simulink model "ad9361_rx_rates"  (R2017b)
settings: Solver=ode23  StartTime=0.0  StopTime=inf  RelTol=1e-3  EnableMultiTasking=on
PreLoadFcn:
  | SampleTime_rx = 1.302083333333333334e-7;
  | 
  | ad9361_preload(bdroot,'rx')
undefined symbols (not defined in the file or in its folder): magnitude, var
libraries: dspsrcs4 x8, dspmathops x6, dsparch4 x4, ad9361_models x1
CloseFcn:
  | clear ad9361_rx_hm1Filt ad9361_rx_hm2Filt;
  | clear ad9361_rx_hm3Filt ad9361_rx_hm4Filt;
  | clear SampleTime_rx;
settings Model: Creator=The MathWorks Inc.  LastModifiedBy=ppradhan
settings DataIOCC: ExternalInput=txWaveform  SaveFormat=StructureWithTime  SaveOutput=off  SignalLogging=off  DSMLogging=off  SaveTime=off  OutputSaveName=rx
settings OptimizationCC: DefaultParameterBehavior=Inlined  InlineInvariantSignals=on  EfficientMapNaN2IntZero=off  LifeSpan=inf  SimCompilerOptimization=on
settings DebuggingCC: ReadBeforeWriteMsg=DisableAll  WriteAfterWriteMsg=DisableAll  WriteAfterReadMsg=DisableAll  UnderspecifiedInitializationDetection=Classic  MergeDetectMultiDrivingBlocksExec=none  SolverPrmCheckMsg=warning  InheritedTsInSrcMsg=none  MultiTaskDSMMsg=none  IntegerOverflowMsg=none  AllowSymbolicDim=off  SFUnexpectedBacktrackingDiag=warning  SFNoUnconditionalDefaultTransitionDiag=none  SFUndirectedBroadcastEventsDiag=none  SFExecutionAtInitializationDiag=none  IntegerSaturationMsg=none
settings HardwareCC: ProdBitPerPointer=32  ProdBitPerSizeT=32  ProdBitPerPtrDiffT=32  ProdLargestAtomicFloat=None  ProdIntDivRoundTo=Undefined  ProdEndianess=Unspecified  ProdWordSize=32  ProdHWDeviceType=32-bit Generic  TargetBitPerPointer=64  TargetBitPerSizeT=64  TargetBitPerPtrDiffT=64  TargetLongLongMode=on  TargetIntDivRoundTo=Zero  TargetEndianess=LittleEndian  TargetWordSize=64  TargetHWDeviceType=MATLAB Host  ProdEqTarget=off
settings ModelReferenceCC: UpdateModelReferenceTargets=IfOutOfDate  PropagateSignalLabelsOutOfModel=off
settings SFSimCC: SFSimEcho=off
settings CodeAppCC: MaxIdLength=128  StateflowObjectComments=on
settings GRTTargetCC: TargetLangStandard=C89/C90 (ANSI)  GeneratePreprocessorConditionals=Disable all  CombineOutputUpdateFcns=off  GRTInterface=on
settings ConfigComp: CovMetricSettings=dw  CovHtmlReporting=on  CovSaveCumulativeToWorkspaceVar=on  CovSaveSingleToWorkspaceVar=on  CovExternalEMLEnable=off  CovSFcnEnable=off
settings SimscapeCC: ExplicitSolverDiagnosticOptions=none

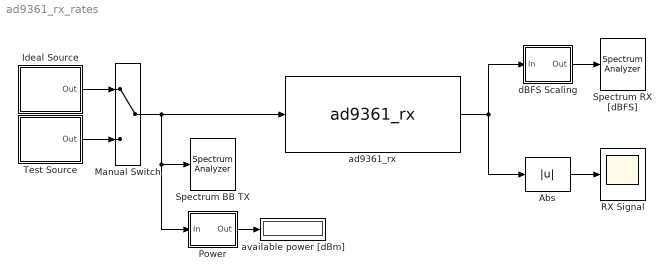
== system ad9361_rx_rates ==
  Abs : Abs
  Ideal Source : Subsystem  mask{Sel=Single CW tone, CW=1e6, Pow=-70, Tstep=1.302083333333333e-07, Ovs=4}
      mask prompts: Sel "Select source"; CW "Frequency (Hz)"; Pow "Power (dBm)"; Tstep "Sample time (s)"; Ovs "Oversampling"
      mask TypeOptions Sel: CW + 1MHz tone | Single CW tone | Dual CW tone
      mask DialogControl DescGroupVar Prompt: Ideal Test Source
  Manual Switch : ManualSwitch
  "Power  " : Subsystem  mask{R=50}
      mask prompts: R "Reference Impedance [Ohm]"
      mask DialogControl DescGroupVar Prompt: Power Meter
  RX Signal : Scope
  Spectrum BB TX : SpectrumAnalyzer
  Spectrum RX [dBFS] : SpectrumAnalyzer
  Test Source : Subsystem  mask{TestSigType=5MHz LTE-like test signal, RxCustVector=complex(rand(1000,1), rand(1000,1)), Tstep=1.302083333333333e-07, OverSample=4, LTE_Pow=-50, hasBlockerCW=off, CW_Blocker_Freq=3e6, CW_Blocker_Pow=-20, hasBlockerLTE=off, LTE_Blocker_OffsetFreq=3e6, LTE_Blocker_Pow=-30}
      mask prompts: TestSigType "Test signal"; RxCustVector "Custom test vector complex data (I, Q)"; Tstep "Sample time (s)"; OverSample "Oversampling"; LTE_Pow "Power (dBm)"; hasBlockerCW "CW blocker"; CW_Blocker_Freq "Frequency CW blocker (Hz)"; CW_Blocker_Pow "Power CW blocker (dBm)"; hasBlockerLTE "LTE-like blocker"; LTE_Blocker_OffsetFreq "Frequency offset LTE-like blocker (Hz)"; LTE_Blocker_Pow "Power LTE-like blocker (dBm)"
      mask init:
      | load ad9361_LTE_data;
      | load ad9361_LTE_blocker;
      | 
      | if strcmpi(TestSigType,'5MHz LTE-like test signal')
      |     tx = tx5;
      |     tx_bl = tx5_bl;
      |     SampleTime_rx = 1/info5.SamplingRate;
      |     LTE = 5;
      | elseif strcmpi(TestSigType,'10MHz LTE-like test signal')
      |     tx = tx10;
      |     tx_bl = tx10_bl;
      |     LTE = 10;
      |     SampleTime_rx = 1/info10.SamplingRate;
      | elseif strcmpi(TestSigType,'20MHz LTE-like test signal')
      |     tx = tx20;
      |     tx_bl = tx20_bl;
      |     LTE = 20;
      |     SampleTime_rx = 1/info20.SamplingRate;
      | elseif strcmpi(TestSigType,'Custom Signal (LTE blocker NOT allowed)')
      |     LTE = 0;
      |     tx = RxCustVector;
      |     tx_bl = RxCustVector;
      |     SampleTime_rx = str2num(get_param(gcb,'Tstep'));
      | else
      |     error(message('simrf:simrfad9361:UnknownTestSig',gcb,TestSigType));
      | end
      | 
      | if ~any(strcmpi(get_param(bdroot(gcb), 'SimulationStatus'),             ...
      |             {'running' 'paused'}))
      |   set_param(gcb,'Tstep',num2str(SampleTime_rx,16));
      |   idlSrc = [bdroot '/Ideal Source'];
      |   set_param(idlSrc,'Tstep',num2str(SampleTime_rx,16));
      |   if ~strcmp(TestSigType,'Custom signal (LTE blocker NOT allowed)')
      |     assignin('base', 'SampleTime_rx', SampleTime_rx);
      |   end
      |   p = Simulink.Mask.get(gcb);
      |   p.Parameters(3).Value = num2str(SampleTime_rx,16);
      | end
      mask TypeOptions TestSigType: 5MHz LTE-like test signal | 10MHz LTE-like test signal | 20MHz LTE-like test signal | Custom Signal (LTE blocker NOT allowed)
      mask Callback TestSigType:
      | % Set Mask visibilites and enables
      | ad9361_rx_mask_callbacks(gcb,'TestSigType')
      mask Callback hasBlockerCW:
      | % Set Mask visibilites and enables
      | ad9361_rx_mask_callbacks(gcb,'hasBlockerCW')
      mask Callback hasBlockerLTE:
      | % Set Mask visibilites and enables
      | ad9361_rx_mask_callbacks(gcb,'hasBlockerLTE')
      mask DialogControl DescGroupVar Prompt: Test Source RX
  ad9361_rx : ad9361_models/ad9361_rx  TestSignal=5MHz LTE  LO=2e9  RF=2e9  Trf=1/(4*7.68e6)
      settings: SourceProductName=RF Blockset Models for Analog Devices RF Transceivers
  available power [dBm] : Display
  dBFS Scaling : Subsystem
  wires:
  Test Source/1(Out) -> Manual Switch/2
  Ideal Source/1(Out) -> Manual Switch/1
  Manual Switch/1 -> ad9361_rx/1, Spectrum BB TX/1, "Power  "/1(In)
  "Power  "/1(Out) -> available power [dBm]/1
  dBFS Scaling/1(Out) -> Spectrum RX [dBFS]/1
  ad9361_rx/1 -> Abs/1, dBFS Scaling/1(In)
  Abs/1 -> RX Signal/1

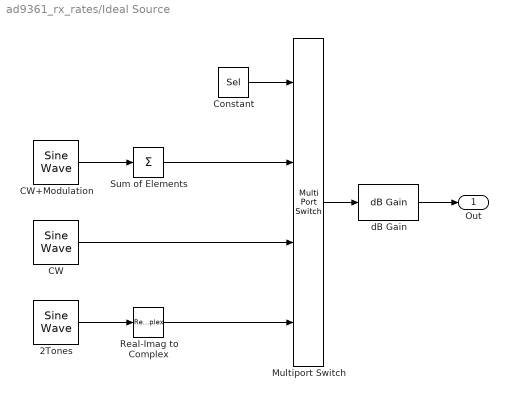
== system ad9361_rx_rates/Ideal Source ==
  2Tones : dspsrcs4/Sine Wave  Amplitude=sqrt(2)  Frequency=CW/2  Phase=0  SampleMode=Discrete  OutComplex=Real  CompMethod=Trigonometric fcn  TableSize=Speed  SampleTime=Tstep/Ovs  SamplesPerFrame=1  ResetState=Restart at time zero  OutputFrames=on  dataType=double  wordLen=16  udDataType=sfix(16)  fracBitsMode=Best precision  numFracBits=15  OutDataTypeStr=double  LastOutDataTypeStr=double
  CW : dspsrcs4/Sine Wave  Amplitude=1  Frequency=CW  Phase=0  SampleMode=Discrete  OutComplex=Complex  CompMethod=Trigonometric fcn  TableSize=Speed  SampleTime=Tstep/Ovs  SamplesPerFrame=1  ResetState=Restart at time zero  OutputFrames=on  dataType=double  wordLen=16  udDataType=sfix(16)  fracBitsMode=Best precision  numFracBits=15  OutDataTypeStr=double  LastOutDataTypeStr=double
  CW+Modulation : dspsrcs4/Sine Wave  Amplitude=[1; 1]/sqrt(2)  Frequency=[CW; 1e6]  Phase=[0; 0]  SampleMode=Discrete  OutComplex=Complex  CompMethod=Trigonometric fcn  TableSize=Speed  SampleTime=Tstep/Ovs  SamplesPerFrame=1  ResetState=Restart at time zero  OutputFrames=on  dataType=double  wordLen=16  udDataType=sfix(16)  fracBitsMode=Best precision  numFracBits=15  OutDataTypeStr=double  LastOutDataTypeStr=double
  Constant : Constant  Value=Sel  SampleTime=Tstep/Ovs
  Multiport Switch : MultiPortSwitch
  Real-Imag to Complex : RealImagToComplex  Input=Real
  Sum of Elements : Sum  Inputs=+
  dB Gain : dspmathops/dB Gain  dB=Pow-30+20*log10(sqrt(50))  intype=Amplitude
      settings: SourceProductName=DSP System Toolbox  SourceProductBaseCode=DS
  Out : Outport
  wires:
  dB Gain/1 -> Out/1
  Multiport Switch/1 -> dB Gain/1
  Real-Imag to Complex/1 -> Multiport Switch/4
  Constant/1 -> Multiport Switch/1
  2Tones/1 -> Real-Imag to Complex/1
  CW/1 -> Multiport Switch/3
  Sum of Elements/1 -> Multiport Switch/2
  CW+Modulation/1 -> Sum of Elements/1

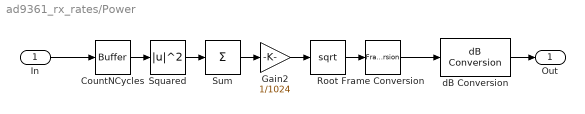
== system ad9361_rx_rates/Power   ==
  In : Inport
  CountNCycles : Buffer  N=1024
  Frame Conversion : FrameConversion  InheritSamplingMode=off  OutFrame=Sample-based
  Gain2 : Gain  Gain=1/1024
  Root : Sqrt  SaturateOnIntegerOverflow=on
  Squared : Math  Operator=magnitude^2  SaturateOnIntegerOverflow=on
  Sum : Sum  Inputs=+
  dB Conversion : dspmathops/dB Conversion  dBtype=dBm  intype=Amplitude  R=R  fuzz=on
      settings: SourceProductName=DSP System Toolbox
  Out : Outport
  wires:
  dB Conversion/1 -> Out/1
  In/1 -> CountNCycles/1
  Frame Conversion/1 -> dB Conversion/1
  CountNCycles/1 -> Squared/1
  Squared/1 -> Sum/1
  Sum/1 -> Gain2/1
  Root/1 -> Frame Conversion/1
  Gain2/1 -> Root/1

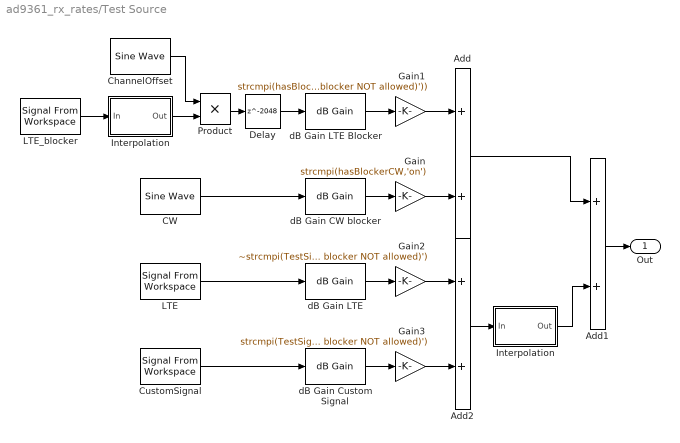
== system ad9361_rx_rates/Test Source ==
  Add : Sum
  Add1 : Sum
  Add2 : Sum
  CW : dspsrcs4/Sine Wave  Amplitude=1  Frequency=CW_Blocker_Freq  Phase=0  SampleMode=Discrete  OutComplex=Complex  CompMethod=Trigonometric fcn  TableSize=Speed  SampleTime=Tstep/OverSample  SamplesPerFrame=1  ResetState=Restart at time zero  OutputFrames=on  dataType=double  wordLen=16  udDataType=sfix(16)  fracBitsMode=Best precision  numFracBits=15  OutDataTypeStr=double  LastOutDataTypeStr=double
  ChannelOffset : dspsrcs4/Sine Wave  Amplitude=1  Frequency=LTE_Blocker_OffsetFreq  Phase=0  SampleMode=Discrete  OutComplex=Complex  CompMethod=Trigonometric fcn  TableSize=Speed  SampleTime=Tstep/OverSample  SamplesPerFrame=1  ResetState=Restart at time zero  OutputFrames=on  dataType=double  wordLen=16  udDataType=sfix(16)  fracBitsMode=Best precision  numFracBits=15  OutDataTypeStr=double  LastOutDataTypeStr=double
  CustomSignal : dspsrcs4/Signal From Workspace  X=repmat(tx,10,1)  Ts=Tstep  nsamps=1  OutputAfterFinalValue=Setting to zero  ignoreOrWarnInputAndFrameLengths=off  OutputFrames=on
  Delay : Delay  DelayLength=2048
  Gain : Gain  Gain=strcmpi(hasBlockerCW,'on')
  Gain1 : Gain  Gain=strcmpi(hasBlockerLTE,'on')&&(~strcmpi(TestSigType,'Custom Signal (LTE blocker NOT allowed)'))
  Gain2 : Gain  Gain=~strcmpi(TestSigType,'Custom Signal (LTE blocker NOT allowed)')
  Gain3 : Gain  Gain=strcmpi(TestSigType,'Custom Signal (LTE blocker NOT allowed)')
  Interpolation : Subsystem
  "Interpolation " : Subsystem
  LTE : dspsrcs4/Signal From Workspace  X=repmat(tx,10,1)  Ts=Tstep  nsamps=1  OutputAfterFinalValue=Setting to zero  ignoreOrWarnInputAndFrameLengths=off  OutputFrames=on
  LTE_blocker : dspsrcs4/Signal From Workspace  X=repmat(tx_bl,10,1)  Ts=Tstep  nsamps=1  OutputAfterFinalValue=Setting to zero  ignoreOrWarnInputAndFrameLengths=off  OutputFrames=on
  Product : Product
  dB Gain CW blocker : dspmathops/dB Gain  dB=CW_Blocker_Pow-30+20*log10(sqrt(50))  intype=Amplitude
      settings: SourceProductName=DSP System Toolbox  SourceProductBaseCode=DS
  dB Gain Custom Signal : dspmathops/dB Gain  dB=LTE_Pow - (10*log10(var(tx))+30)+20*log10(sqrt(50))  intype=Amplitude
      settings: SourceProductName=DSP System Toolbox  SourceProductBaseCode=DS
  dB Gain LTE : dspmathops/dB Gain  dB=LTE_Pow-10*log10(var(tx))-12  intype=Amplitude
      settings: SourceProductName=DSP System Toolbox  SourceProductBaseCode=DS
  dB Gain LTE Blocker : dspmathops/dB Gain  dB=LTE_Blocker_Pow-10*log10(var(tx_bl))-12  intype=Amplitude
      settings: SourceProductName=DSP System Toolbox  SourceProductBaseCode=DS
  Out : Outport
  wires:
  dB Gain CW blocker/1 -> Gain/1
  Gain/1 -> Add/2
  LTE/1 -> dB Gain LTE/1
  LTE_blocker/1 -> Interpolation/1(In)
  Gain1/1 -> Add/1
  Interpolation/1(Out) -> Product/2
  Product/1 -> Delay/1
  ChannelOffset/1 -> Product/1
  dB Gain LTE/1 -> Gain2/1
  dB Gain LTE Blocker/1 -> Gain1/1
  Gain2/1 -> Add2/1
  dB Gain Custom Signal/1 -> Gain3/1
  Gain3/1 -> Add2/2
  Delay/1 -> dB Gain LTE Blocker/1
  CustomSignal/1 -> dB Gain Custom Signal/1
  Add2/1 -> "Interpolation "/1(In)
  Add/1 -> Add1/1
  "Interpolation "/1(Out) -> Add1/2
  Add1/1 -> Out/1
  CW/1 -> dB Gain CW blocker/1

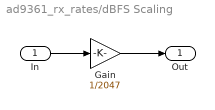
== system ad9361_rx_rates/dBFS Scaling ==
  In : Inport
  Gain : Gain  Gain=1/2047
  Out : Outport
  wires:
  In/1 -> Gain/1
  Gain/1 -> Out/1

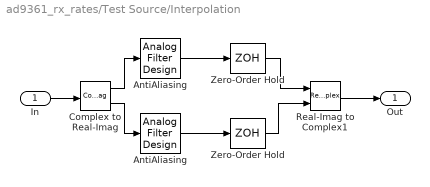
== system ad9361_rx_rates/Test Source/Interpolation ==
  In : Inport
  AntiAliasing : dsparch4/Analog Filter Design  method=Elliptic  filttype=Lowpass  N=8  Wlo=2*pi/(2*Tstep)  Whi=80  Rp=0.1  Rs=80
  "AntiAliasing " : dsparch4/Analog Filter Design  method=Elliptic  filttype=Lowpass  N=8  Wlo=2*pi/(2*Tstep)  Whi=80  Rp=0.1  Rs=80
  Complex to Real-Imag : ComplexToRealImag
  Real-Imag to Complex1 : RealImagToComplex
  Zero-Order Hold : ZeroOrderHold  SampleTime=Tstep/OverSample
  "Zero-Order Hold " : ZeroOrderHold  SampleTime=Tstep/OverSample
  Out : Outport
  wires:
  "Zero-Order Hold "/1 -> Real-Imag to Complex1/2
  Complex to Real-Imag/2 -> "AntiAliasing "/1
  Complex to Real-Imag/1 -> AntiAliasing/1
  In/1 -> Complex to Real-Imag/1
  Zero-Order Hold/1 -> Real-Imag to Complex1/1
  AntiAliasing/1 -> Zero-Order Hold/1
  "AntiAliasing "/1 -> "Zero-Order Hold "/1
  Real-Imag to Complex1/1 -> Out/1

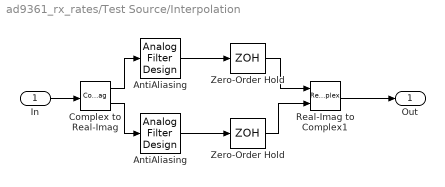
== system ad9361_rx_rates/Test Source/Interpolation  ==
  In : Inport
  AntiAliasing : dsparch4/Analog Filter Design  method=Elliptic  filttype=Lowpass  N=8  Wlo=2*pi/(2*Tstep)  Whi=80  Rp=0.1  Rs=80
  "AntiAliasing " : dsparch4/Analog Filter Design  method=Elliptic  filttype=Lowpass  N=8  Wlo=2*pi/(2*Tstep)  Whi=80  Rp=0.1  Rs=80
  Complex to Real-Imag : ComplexToRealImag
  Real-Imag to Complex1 : RealImagToComplex
  Zero-Order Hold : ZeroOrderHold  SampleTime=Tstep/OverSample
  "Zero-Order Hold " : ZeroOrderHold  SampleTime=Tstep/OverSample
  Out : Outport
  wires:
  "Zero-Order Hold "/1 -> Real-Imag to Complex1/2
  Complex to Real-Imag/2 -> "AntiAliasing "/1
  Complex to Real-Imag/1 -> AntiAliasing/1
  In/1 -> Complex to Real-Imag/1
  Zero-Order Hold/1 -> Real-Imag to Complex1/1
  AntiAliasing/1 -> Zero-Order Hold/1
  "AntiAliasing "/1 -> "Zero-Order Hold "/1
  Real-Imag to Complex1/1 -> Out/1
